simulink model "single_phase_multilevel"  (R2025a)
settings: Solver=ode1be  StartTime=0.0  StopTime=simlength  FixedStep=tc  RelTol=1e-3
values from neighbouring files (symbols this model uses):
  Vfc1_base = Udc/5    [plotting_results.m]    (also in plotting_results_hf.m)
  Vfc2_base = 2*Vfc1_base    [plotting_results.m]    (also in plotting_results_hf.m)
  Vfc3_base = 3*Vfc1_base    [plotting_results.m]    (also in plotting_results_hf.m)
  Vfc4_base = 4*Vfc1_base    [plotting_results.m]    (also in plotting_results_hf.m)
undefined symbols (not defined in the file or in its folder): DThs_init, g0_4Hz, g1_4Hz, I_FS, kalman_omega, kalman_theta, ki_i_inv, ki_v_inv, kp_i_inv, kp_v_inv, Lconn, LFu1, m_dead_time, m_duty_open_loop, magnitude, n1, n10, omega_ref, phase_shift_mod11, phase_shift_mod21, phase_shift_mod31, phase_shift_mod41, phase_shift_mod51, precharge_off, q1kalman, q2kalman, Rbalance, Rconn, RFu, Rg_off, Rg_on, Rkalman, RLFu1, Rprecharge, Tambient, tc, time_pwm_enable, tPWM, ts, V_FS, VCFc_5_init, Vgate_base, weigth
libraries: fl_lib x281, nesl_utility x97, ee_lib x15, simulink x1
(part 4 of 6)

== system single_phase_multilevel/vi_ctrl/modulator1 ==
  m : Inport
  Constant7 : Constant  Value=-m_dead_time
  Constant8 : Constant  Value=m_dead_time
  Data Type Conversion : DataTypeConversion  OutDataTypeStr=double  SaturateOnIntegerOverflow=off  RndMeth=Floor
  Data Type Conversion1 : DataTypeConversion  OutDataTypeStr=double  SaturateOnIntegerOverflow=off  RndMeth=Floor
  Gain : Gain  Gain=Vgate_base
  Gain1 : Gain  Gain=Vgate_base
  Relational Operator : RelationalOperator  Operator=<=
  Relational Operator1 : RelationalOperator  Operator=<=
  Sum1 : Sum  Inputs=|++
  Sum2 : Sum  Inputs=++|
  g11/g12 : Scope  NumInputPorts=2
      settings: SampleTime=tc  ActiveDisplayYMinimum=-0.12499999999999997  ActiveDisplayYMaximum=1.125
  triangle_1 : Subsystem
  g11 : Outport
  g12 : Outport  Port=2
  tag scope: carry_g11=global
  wires:
  m/1 -> Sum1/2, Sum2/1
  Relational Operator/1 -> Data Type Conversion/1
  Relational Operator1/1 -> Data Type Conversion1/1
  Data Type Conversion/1 -> g11/g12/1, Gain/1
  triangle_1/1(carry_mod11) -> Relational Operator1/2, Relational Operator/1, [carry_g11]
  Constant7/1 -> Sum1/1
  Data Type Conversion1/1 -> g11/g12/2, Gain1/1
  Sum2/1 -> Relational Operator1/1
  Constant8/1 -> Sum2/2
  Sum1/1 -> Relational Operator/2
  Gain/1 -> g11/1
  Gain1/1 -> g12/1

== system single_phase_multilevel/vi_ctrl/modulator2 ==
  m : Inport
  Constant7 : Constant  Value=-m_dead_time
  Constant8 : Constant  Value=m_dead_time
  Data Type Conversion : DataTypeConversion  OutDataTypeStr=double  SaturateOnIntegerOverflow=off  RndMeth=Floor
  Data Type Conversion1 : DataTypeConversion  OutDataTypeStr=double  SaturateOnIntegerOverflow=off  RndMeth=Floor
  Gain : Gain  Gain=Vgate_base
  Gain1 : Gain  Gain=Vgate_base
  Relational Operator : RelationalOperator  Operator=<=
  Relational Operator1 : RelationalOperator  Operator=<=
  Sum1 : Sum  Inputs=|++
  Sum2 : Sum  Inputs=++|
  triangle_1 : Subsystem
  g21 : Outport
  g22 : Outport  Port=2
  tag scope: carry_g21=global
  wires:
  Sum1/1 -> Relational Operator/2
  Constant8/1 -> Sum2/2
  Sum2/1 -> Relational Operator1/1
  Data Type Conversion1/1 -> Gain1/1
  Constant7/1 -> Sum1/1
  triangle_1/1(carry_mod21) -> [carry_g21], Relational Operator1/2, Relational Operator/1
  Data Type Conversion/1 -> Gain/1
  Relational Operator1/1 -> Data Type Conversion1/1
  Relational Operator/1 -> Data Type Conversion/1
  m/1 -> Sum2/1, Sum1/2
  Gain/1 -> g21/1
  Gain1/1 -> g22/1

== system single_phase_multilevel/vi_ctrl/modulator3 ==
  m : Inport
  Constant7 : Constant  Value=-m_dead_time
  Constant8 : Constant  Value=m_dead_time
  Data Type Conversion : DataTypeConversion  OutDataTypeStr=double  SaturateOnIntegerOverflow=off  RndMeth=Floor
  Data Type Conversion1 : DataTypeConversion  OutDataTypeStr=double  SaturateOnIntegerOverflow=off  RndMeth=Floor
  Gain : Gain  Gain=Vgate_base
  Gain1 : Gain  Gain=Vgate_base
  Relational Operator : RelationalOperator  Operator=<=
  Relational Operator1 : RelationalOperator  Operator=<=
  Sum1 : Sum  Inputs=|++
  Sum2 : Sum  Inputs=++|
  triangle_1 : Subsystem
  g21 : Outport
  g22 : Outport  Port=2
  tag scope: carry_g31=global
  wires:
  m/1 -> Sum1/2, Sum2/1
  Relational Operator/1 -> Data Type Conversion/1
  Relational Operator1/1 -> Data Type Conversion1/1
  Data Type Conversion/1 -> Gain/1
  triangle_1/1(carry_mod21) -> Relational Operator/1, Relational Operator1/2, [carry_g31]
  Constant7/1 -> Sum1/1
  Data Type Conversion1/1 -> Gain1/1
  Sum2/1 -> Relational Operator1/1
  Constant8/1 -> Sum2/2
  Sum1/1 -> Relational Operator/2
  Gain/1 -> g21/1
  Gain1/1 -> g22/1

== system single_phase_multilevel/vi_ctrl/modulator4 ==
  m : Inport
  Constant7 : Constant  Value=-m_dead_time
  Constant8 : Constant  Value=m_dead_time
  Data Type Conversion : DataTypeConversion  OutDataTypeStr=double  SaturateOnIntegerOverflow=off  RndMeth=Floor
  Data Type Conversion1 : DataTypeConversion  OutDataTypeStr=double  SaturateOnIntegerOverflow=off  RndMeth=Floor
  Gain : Gain  Gain=Vgate_base
  Gain1 : Gain  Gain=Vgate_base
  Relational Operator : RelationalOperator  Operator=<=
  Relational Operator1 : RelationalOperator  Operator=<=
  Sum1 : Sum  Inputs=|++
  Sum2 : Sum  Inputs=++|
  triangle_1 : Subsystem
  g21 : Outport
  g22 : Outport  Port=2
  tag scope: carry_g41=global
  wires:
  m/1 -> Sum1/2, Sum2/1
  Relational Operator/1 -> Data Type Conversion/1
  Relational Operator1/1 -> Data Type Conversion1/1
  Data Type Conversion/1 -> Gain/1
  triangle_1/1(carry_mod21) -> Relational Operator/1, Relational Operator1/2, [carry_g41]
  Constant7/1 -> Sum1/1
  Data Type Conversion1/1 -> Gain1/1
  Sum2/1 -> Relational Operator1/1
  Constant8/1 -> Sum2/2
  Sum1/1 -> Relational Operator/2
  Gain/1 -> g21/1
  Gain1/1 -> g22/1

== system single_phase_multilevel/vi_ctrl/modulator5 ==
  m : Inport
  Constant7 : Constant  Value=-m_dead_time
  Constant8 : Constant  Value=m_dead_time
  Data Type Conversion : DataTypeConversion  OutDataTypeStr=double  SaturateOnIntegerOverflow=off  RndMeth=Floor
  Data Type Conversion1 : DataTypeConversion  OutDataTypeStr=double  SaturateOnIntegerOverflow=off  RndMeth=Floor
  Gain : Gain  Gain=Vgate_base
  Gain1 : Gain  Gain=Vgate_base
  Relational Operator : RelationalOperator  Operator=<=
  Relational Operator1 : RelationalOperator  Operator=<=
  Sum1 : Sum  Inputs=|++
  Sum2 : Sum  Inputs=++|
  triangle_1 : Subsystem
  g21 : Outport
  g22 : Outport  Port=2
  tag scope: carry_g51=global
  wires:
  Sum1/1 -> Relational Operator/2
  Constant8/1 -> Sum2/2
  Sum2/1 -> Relational Operator1/1
  Data Type Conversion1/1 -> Gain1/1
  Constant7/1 -> Sum1/1
  triangle_1/1(carry_mod21) -> [carry_g51], Relational Operator1/2, Relational Operator/1
  Data Type Conversion/1 -> Gain/1
  Relational Operator1/1 -> Data Type Conversion1/1
  Relational Operator/1 -> Data Type Conversion/1
  m/1 -> Sum2/1, Sum1/2
  Gain/1 -> g21/1
  Gain1/1 -> g22/1

== system single_phase_multilevel/vi_ctrl/pre-charge ==
  dm_in : Inport
  Ramp : simulink/Sources/Ramp  slope=-1  start=0  InitialOutput=0.5
  Saturation : Saturate  UpperLimit=0.25  LowerLimit=0
  Step1 : Step  Time=time_pwm_enable  SampleTime=0
  Switch : Switch  Criteria=u2 > Threshold  Threshold=0.5  SaturateOnIntegerOverflow=off  InputSameDT=off
  dm_out : Outport
  wires:
  Switch/1 -> dm_out/1
  ? -> Saturation/1
  Saturation/1 -> Switch/3
  dm_in/1 -> Switch/1
  Step1/1 -> Switch/2

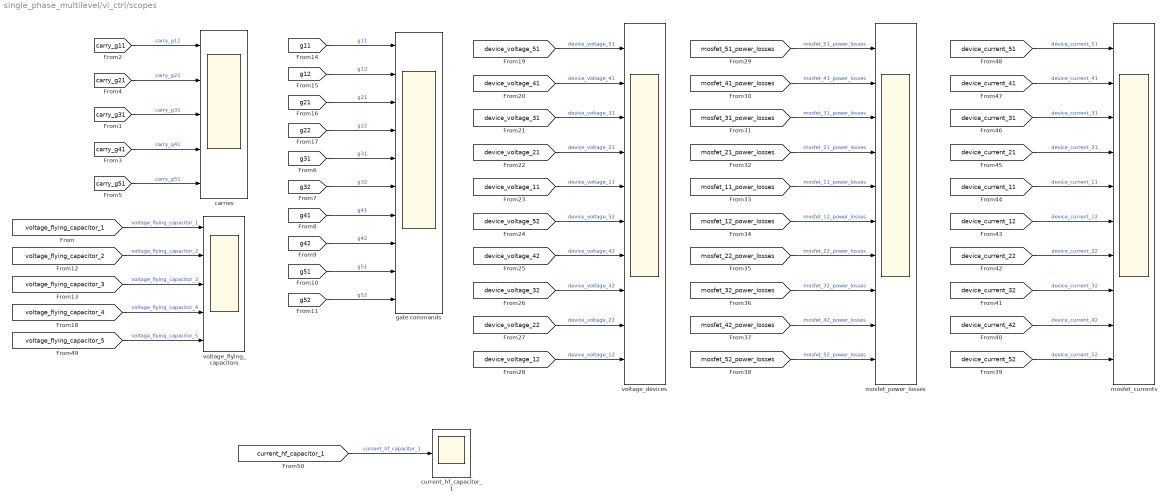
== system single_phase_multilevel/vi_ctrl/scopes ==
  carries : Scope  NumInputPorts=5
      settings: SampleTime=tc  ActiveDisplayYMinimum=-1.64662  ActiveDisplayYMaximum=1.23308  DataLoggingVariableName=ScopeData2
  current_hf_capacitor_1 : Scope
      settings: SampleTime=tc  ActiveDisplayYMinimum=-3.192455025047797  ActiveDisplayYMaximum=2.3538130408116107
  gate commands : Scope  NumInputPorts=10
      settings: SampleTime=tc  ActiveDisplayYMinimum=-1.875  ActiveDisplayYMaximum=16.875  DataLoggingVariableName=ScopeData3
  mosfet_currents : Scope  NumInputPorts=10
      settings: SampleTime=tc  ActiveDisplayYMinimum=-162.1625098340769  ActiveDisplayYMaximum=1459.4625889259892
  mosfet_power_losses : Scope  NumInputPorts=10
      settings: SampleTime=tc  ActiveDisplayYMinimum=-0.01246  ActiveDisplayYMaximum=0.84421  DataLoggingVariableName=ScopeData2
  voltage_devices : Scope  NumInputPorts=10
      settings: SampleTime=tc  ActiveDisplayYMinimum=1.7653686212392756  ActiveDisplayYMaximum=403.40848662720771  DataLoggingVariableName=ScopeData3
  voltage_flying_capacitors : Scope  NumInputPorts=5
      settings: SampleTime=tc  ActiveDisplayYMinimum=-145.59590564608663  ActiveDisplayYMaximum=3675.5801398737103
  wires:
  [carry_g51] -> carries/5  "carry_g51"
  [g12] -> gate commands/2  "g12"
  [g11] -> gate commands/1  "g11"
  [g41] -> gate commands/7  "g41"
  [carry_g41] -> carries/4  "carry_g41"
  [g52] -> gate commands/10  "g52"
  [carry_g31] -> carries/3  "carry_g31"
  [g31] -> gate commands/5  "g31"
  [g21] -> gate commands/3  "g21"
  [voltage_flying_capacitor_4] -> voltage_flying_capacitors/4  "voltage_flying_capacitor_4"
  [carry_g11] -> carries/1  "carry_g11"
  [g42] -> gate commands/8  "g42"
  [voltage_flying_capacitor_1] -> voltage_flying_capacitors/1  "voltage_flying_capacitor_1"
  [g22] -> gate commands/4  "g22"
  [g32] -> gate commands/6  "g32"
  [g51] -> gate commands/9  "g51"
  [voltage_flying_capacitor_3] -> voltage_flying_capacitors/3  "voltage_flying_capacitor_3"
  [voltage_flying_capacitor_2] -> voltage_flying_capacitors/2  "voltage_flying_capacitor_2"
  [carry_g21] -> carries/2  "carry_g21"
  [device_current_11] -> mosfet_currents/5  "device_current_11"
  [mosfet_12_power_losses] -> mosfet_power_losses/6  "mosfet_12_power_losses"
  [device_current_32] -> mosfet_currents/8  "device_current_32"
  [mosfet_21_power_losses] -> mosfet_power_losses/4  "mosfet_21_power_losses"
  [device_voltage_42] -> voltage_devices/7  "device_voltage_42"
  [device_voltage_21] -> voltage_devices/4  "device_voltage_21"
  [device_current_12] -> mosfet_currents/6  "device_current_12"
  [device_voltage_52] -> voltage_devices/6  "device_voltage_52"
  [device_voltage_41] -> voltage_devices/2  "device_voltage_41"
  [device_voltage_51] -> voltage_devices/1  "device_voltage_51"
  [device_voltage_11] -> voltage_devices/5  "device_voltage_11"
  [mosfet_31_power_losses] -> mosfet_power_losses/3  "mosfet_31_power_losses"
  [device_voltage_22] -> voltage_devices/9  "device_voltage_22"
  [device_current_51] -> mosfet_currents/1  "device_current_51"
  [device_current_41] -> mosfet_currents/2  "device_current_41"
  [device_voltage_12] -> voltage_devices/10  "device_voltage_12"
  [device_voltage_32] -> voltage_devices/8  "device_voltage_32"
  [device_voltage_31] -> voltage_devices/3  "device_voltage_31"
  [mosfet_32_power_losses] -> mosfet_power_losses/8  "mosfet_32_power_losses"
  [mosfet_11_power_losses] -> mosfet_power_losses/5  "mosfet_11_power_losses"
  [mosfet_51_power_losses] -> mosfet_power_losses/1  "mosfet_51_power_losses"
  [mosfet_41_power_losses] -> mosfet_power_losses/2  "mosfet_41_power_losses"
  [mosfet_42_power_losses] -> mosfet_power_losses/9  "mosfet_42_power_losses"
  [mosfet_52_power_losses] -> mosfet_power_losses/10  "mosfet_52_power_losses"
  [mosfet_22_power_losses] -> mosfet_power_losses/7  "mosfet_22_power_losses"
  [device_current_42] -> mosfet_currents/9  "device_current_42"
  [device_current_31] -> mosfet_currents/3  "device_current_31"
  [device_current_22] -> mosfet_currents/7  "device_current_22"
  [device_current_21] -> mosfet_currents/4  "device_current_21"
  [device_current_52] -> mosfet_currents/10  "device_current_52"
  [voltage_flying_capacitor_5] -> voltage_flying_capacitors/5  "voltage_flying_capacitor_5"
  [current_hf_capacitor_1] -> current_hf_capacitor_1/1  "current_hf_capacitor_1"

== system single_phase_multilevel/vi_ctrl/single_phase_contrl_system ==
  1/Ti2 : Gain  Gain=1/V_FS  SaturateOnIntegerOverflow=on  OutDataTypeStr=Inherit: Same as input  ParamDataTypeStr=Inherit: Same as input
  Constant1 : Constant  Value=0
  Math Function : Math  Operator=magnitude^2
  Math Function1 : Math  Operator=magnitude^2
  Sqrt : Sqrt
  Sum1 : Sum  Inputs=|-+
  Sum2 : Sum  Inputs=+-|
  Sum3 : Sum  Inputs=|++
  Sum4 : Sum  Inputs=|-+
  Zero-Order Hold4 : ZeroOrderHold  SampleTime=ts
  acquisition_and_scaling_current : Subsystem
  acquisition_and_scaling_voltage : Subsystem
  alpha_beta_transformation_i : Subsystem
  alpha_beta_transformation_v : Subsystem
  alphabeta2dq : Subsystem
  dq2alphabeta : Subsystem
  i_alpha_beta : Scope  NumInputPorts=2
      settings: ActiveDisplayYMinimum=-0.6421  ActiveDisplayYMaximum=0.5039
  idq : Scope  NumInputPorts=2
      settings: ActiveDisplayYMinimum=-0.09367  ActiveDisplayYMaximum=0.50142
  inverter current/voltage : Scope  NumInputPorts=3
      settings: SampleTime=tc  ActiveDisplayYMinimum=-1.0984397723811322E-13  ActiveDisplayYMaximum=2.3609927412802815E-14  DataLoggingVariableName=ScopeData2
  phase_gen : Subsystem
  pi_d : Subsystem
  pi_q : Subsystem
  pi_v : Subsystem
  reference_flt : Subsystem
  v_reference : Step  Time=precharge_off  After=230*sqrt(2)  SampleTime=0
  alpha : Outport
  tag scope: uout_magnitude_pu=global, uout_magnitude_pu_ref=global
  wires:
  [inverter_current_output] -> inverter current/voltage/1  "inverter_current_output_modA"
  [inverter_current_output] -> acquisition_and_scaling_current/1(in)
  pi_d/1(Vd_out) -> dq2alphabeta/1(d)
  pi_v/1(i_ref_internal) -> Sum2/1
  Zero-Order Hold4/1 -> reference_flt/1(input)
  alpha_beta_transformation_v/2(beta) -> Math Function1/1
  [inverter_voltage_output] -> inverter current/voltage/2  "inverter_voltager_output_modA"
  alphabeta2dq/2("q ") -> idq/2, Sum1/1
  dq2alphabeta/1(alpha) -> alpha/1
  [inverter_voltage_output] -> acquisition_and_scaling_voltage/1(in)
  Constant1/1 -> Sum1/2
  alphabeta2dq/1("d ") -> idq/1, Sum2/2
  v_reference/1 -> 1/Ti2/1
  Sum4/1 -> pi_v/1(e)
  Math Function1/1 -> Sum3/2
  phase_gen/1(theta) -> alphabeta2dq/3(wt), dq2alphabeta/3(wt)
  1/Ti2/1 -> Zero-Order Hold4/1
  acquisition_and_scaling_current/1(out) -> alpha_beta_transformation_i/1(in)
  Sum3/1 -> Sqrt/1
  Sum1/1 -> pi_q/1(iq_tilde)
  Math Function/1 -> Sum3/1
  Sqrt/1 -> [uout_magnitude_pu], Sum4/1
  pi_q/1(Vd_out) -> dq2alphabeta/2(q)
  Sum2/1 -> pi_d/1(id_tilde)
  alpha_beta_transformation_i/1(alpha) -> i_alpha_beta/1, alphabeta2dq/1(alpha)
  alpha_beta_transformation_i/2(beta) -> i_alpha_beta/2, alphabeta2dq/2(beta)
  acquisition_and_scaling_voltage/1(out) -> alpha_beta_transformation_v/1(in)
  alpha_beta_transformation_v/1(alpha) -> Math Function/1
  [inverter_current_stack] -> inverter current/voltage/3  "inverter_current_stack_modA"
  reference_flt/1(output) -> [uout_magnitude_pu_ref], Sum4/2

== system single_phase_multilevel/flying_capacitor_leg/switch_11/Subsystem ==
  Diode : fl_lib/Electrical/Electrical Elements/Diode  Vf=Vgamma_diode_mosfet V  Ron=Ron_diode_mosfet Ohm  Goff=1e-8 1/Ohm  i_specify=off  i_priority=None  i=0 A  i_nominal_specify=off  i_nominal_value=1  i_nominal_unit=A  v_specify=off  v_priority=None  v=0 V  v_nominal_specify=off  v_nominal_value=1  v_nominal_unit=V
  G3R160MT17D : ee_lib/Semiconductors & Converters/MOSFET (Ideal, Switching)  port_option=ee.enum.controlport.elec  Rds=Rds_on Ohm  Goff=Goff_state_mosfet 1/Ohm  Vth=Vg_threshold V  diode_param=ee.enum.semiconductors.protectionDiode.external  diode_Vf=Vgamma_diode_mosfet V  diode_Ron=Ron_diode_mosfet Ohm  diode_Goff=Goff_state_mosfet 1/Ohm  diode_C=50e-9 F  diode_iRM=-235 A  diode_iF=300 A  diode_idot=-50 A/us  diode_trr_param=ee.enum.converters.diodeReverseParam.trr_factor  diode_trr_factor=3  diode_trr=15 us  diode_Qrr=1500 s*uA  ids_specify=off  ids_priority=None  ids=0 A  ids_nominal_specify=off  ids_nominal_value=1  ids_nominal_unit=A  vds_specify=off  vds_priority=None  vds=0 V  vds_nominal_specify=off  vds_nominal_value=1  vds_nominal_unit=V  vgs_specify=off  vgs_priority=None  vgs=0 V  vgs_nominal_specify=off  vgs_nominal_value=1  vgs_nominal_unit=V  thermal_loss_option=ee.enum.converters.thermalLossOption.constantvalues  Von_data=[0, 1.8, 3.2, 6, 10, 16; 0, 2, 5.5, 9.5, 15, 25] V  Tj=[298.15, 448.15] K  Iout_data=[0, 20, 40, 60, 80, 100] A  Eon_data=[0, 55.04, 124.57, 235.53, 362.12; 0, 71.25, 161.25, 304.88, 468.75] * 1e-6 J  Eoff_data=[0, 18, 30, 56.1, 76.5; 0, 22.5, 37.5, 70.13, 95.63] * 1e-6 J  Eon_data_3D=[zeros(2, 5, 3)] J  Eoff_data_3D=[zeros(2, 5, 3)] J  Tj_loss=[298.15, 448.15] K  Iout_data_loss=[0, 10, 20, 30, 40] A  tabulateWithVds=false  Vds_loss=[0, 150, 300] V  Eon_scalar=Eon J  Eoff_scalar=Eoff J  Voff=Vdc_switching_losses_ref V  Iout_scalar=Ids_switching_losses_ref A  useCurrentFromPreviousCycle=false  useVoltageFromPreviousCycle=false  diodeModelType=ee.enum.converters.diodeModelType.pwl  diodeTableType=ee.enum.diode.tableType.IfMat  diode_ReverseIVType=ee.enum.diode.diodeReverseIV.constant  diode_IfMat=[.07, .12, .19, 1.75, 4.24, 7.32, 11.2; .16, .3, .72, 2.14, 4.02, 6.35, 9.12] A  diode_VfMat=[.9, 1.15, 1.25, 1.5, 1.75, 2.17, 2.6, 2.85; .58, .68, .75, 1.1, 1.38, 1.77, 2.27, 2.7] V  diode_TjVec=[25, 125] degC  diode_VfVec=[.5, .7, .9, 1.3, 1.7, 2.1, 2.5] V  diode_IfVec=[.1, .2, .5, 1, 2, 4, 7, 10] A  diode_IrMat=[1e-06, 2e-06, 5e-06, 1e-05, 2.5e-05, 5e-05, .0001; 2e-06, 5e-06, 1e-05, 4e-05, 8e-05, .0002, .0005] A  diode_VrMat=[10, 100, 200, 250, 300, 325, 350; 10, 70, 160, 220, 270, 300, 320] V  diode_VrVec=[10, 20, 40, 50, 70, 80, 100] V  diode_IrVec=[1e-06, 2e-06, 5e-06, 1e-05, 2e-05, 5e-05, .0001] A  diode_Vr=-600 V  diode_Ls=150 nH  diode_Erec=0.03 J  diode_rec_loss_model=ee.enum.diode.reverseRecoveryModel.fixed  diode_ErecVal=0 J  diode_scaleWithIandV=true  diode_ErecMat=zeros(2, 3) J  diode_TjrecVec=[298.15, 398.15] K  diode_IfrecVec=[.1, 1, 10] A  diode_IrecVal=10 A  diode_VrecVal=10 V  diode_tFilter=1 / 1000 / 100 s  separateThermalPortForDiode=false  thermal_network_parameterization=ee.enum.thermalNetworkTopology.external  Rth=[.03, .2] K/W  Rth_Cauer=[.03, .1, .2] K/W  Rth_Foster=[.03, .2] K/W  thermal_mass_parameterization=ee.enum.thermalNetwork.timeconstant  thermal_mass=[3, 25] J/K  thermal_mass_Cauer=[3, 10, 25] J/K  thermal_mass_Foster=[33, 50] J/K  thermal_time_constant=[.1, 5] s  thermal_time_constant_Cauer=[.1, 1, 5] s  thermal_time_constant_Foster=[1, 10] s  thermal_mass_initial_temperatures=[25, 25] degC  thermal_mass_initial_temperatures_Cauer=[25, 25, 25] degC  junction_thermal_mass=JunctionTermalMass J/K  Tvec_initial_Foster=[25, 25, 25, 25] degC  RthDiode=[.03, .2] K/W  RthCauerDiode=[.03, .1, .2] K/W  RthFosterDiode=[.03, .2] K/W  thermalMassDiode=[3, 25] J/K  thermalMassCauerDiode=[3, 10, 25] J/K  thermalMassFosterDiode=[33, 50] J/K  thermalTauDiode=[.1, 5] s  thermalTauCauerDiode=[.1, 1, 5] s  thermalTauFosterDiode=[1, 10] s  thermalMassInitTempDiode=[25, 25] degC  thermalMassInitTempCauerDiode=[25, 25, 25] degC  junctionthermalMassDiode=0.1 J/K  TVecInitialFosterDiode=[25, 25, 25, 25] degC  no_thermal_network=0  mosfet_junction_temperature_specify=off  mosfet_junction_temperature_priority=None  mosfet_junction_temperature=25 degC  mosfet_junction_temperature_nominal_specify=off  mosfet_junction_temperature_nominal_value=1  mosfet_junction_temperature_nominal_unit=degC  diode_junction_temperature_specify=off  diode_junction_temperature_priority=None  diode_junction_temperature=25 degC  diode_junction_temperature_nominal_specify=off  diode_junction_temperature_nominal_value=1  diode_junction_temperature_nominal_unit=degC  Qj_specify=off  Qj_priority=None  Qj=0 W  Qj_nominal_specify=off  Qj_nominal_value=1  Qj_nominal_unit=W  accumulatedSwitchingLosses_specify=off  accumulatedSwitchingLosses_priority=None  accumulatedSwitchingLosses=0 J
      settings: InternalSimscapePortConfiguration="{\"Bottom\":[],\"Left\":[{\"id\":\"G_elec\",\"label\":\"\",\"type\":\"foundation.electrical.electrical\"},{\"id\":\"H\",\"label\":\"\",\"type\":\"foundation.thermal.thermal\"}],\"Right\":[{\"id\":\"D\",\"label\":\"\",\"type\":\"foundation.electrical.electrical\"},{\"id\":\"S\",\"label\":\"\",\"type\":\"foundation.electrical.electrical\"}],\"Top\":[]}"
  G : PMIOPort  Side=Left
  thermal_port : PMIOPort  Port=2  Side=Left
  D : PMIOPort  Port=3  Side=Left
  S : PMIOPort  Port=4  Side=Right
  connections:
  G3R160MT17D/RConn1 -- Diode/RConn1 -- D/RConn1
  G3R160MT17D/RConn2 -- Diode/LConn1 -- S/RConn1
  G/RConn1 -- G3R160MT17D/LConn1
  G3R160MT17D/LConn2 -- thermal_port/RConn1

== system single_phase_multilevel/flying_capacitor_leg/switch_11/gate_driver ==
  cmd : Inport
  Controlled Voltage Source : fl_lib/Electrical/Electrical Sources/Controlled Voltage Source
  Diode1 : fl_lib/Electrical/Electrical Elements/Diode  Vf=0.6 V  Ron=0.3 Ohm  Goff=1e-8 1/Ohm  i_specify=off  i_priority=None  i=0 A  i_nominal_specify=off  i_nominal_value=1  i_nominal_unit=A  v_specify=off  v_priority=None  v=0 V  v_nominal_specify=off  v_nominal_value=1  v_nominal_unit=V
  Diode2 : fl_lib/Electrical/Electrical Elements/Diode  Vf=0.6 V  Ron=0.3 Ohm  Goff=1e-8 1/Ohm  i_specify=off  i_priority=None  i=0 A  i_nominal_specify=off  i_nominal_value=1  i_nominal_unit=A  v_specify=off  v_priority=None  v=0 V  v_nominal_specify=off  v_nominal_value=1  v_nominal_unit=V
  Resistor : fl_lib/Electrical/Electrical Elements/Resistor  R=Rg_on Ohm  i_specify=off  i_priority=None  i=0 A  i_nominal_specify=off  i_nominal_value=1  i_nominal_unit=A  v_specify=off  v_priority=None  v=0 V  v_nominal_specify=off  v_nominal_value=1  v_nominal_unit=V
  Resistor1 : fl_lib/Electrical/Electrical Elements/Resistor  R=Rg_off Ohm  i_specify=off  i_priority=None  i=0 A  i_nominal_specify=off  i_nominal_value=1  i_nominal_unit=A  v_specify=off  v_priority=None  v=0 V  v_nominal_specify=off  v_nominal_value=1  v_nominal_unit=V
  Simulink-PS Converter : nesl_utility/Simulink-PS Converter  PhysicalDomain=network_engine_domain  SubClassName=ps_input  LeftPortType=input  RightPortType=output  PseudoPeriodic=off  Frequencies=[]  NoiseDistribution=none  NoiseParameters=[]  Unit=V  AffineConversion=off  FilteringAndDerivatives=provide  SimscapeFilterOrder=1  InputFilterTimeConstant=0.001  UdotUserProvided=0
  gate : PMIOPort  Side=Right
  source : PMIOPort  Port=2  Side=Right
  wires:
  cmd/1 -> Simulink-PS Converter/1
  connections:
  Resistor/LConn1 -- Controlled Voltage Source/LConn1 -- Resistor1/LConn1
  Diode2/LConn1 -- Resistor/RConn1
  Controlled Voltage Source/RConn1 -- Simulink-PS Converter/RConn1
  Controlled Voltage Source/RConn2 -- source/RConn1
  Diode1/LConn1 -- gate/RConn1 -- Diode2/RConn1
  Diode1/RConn1 -- Resistor1/RConn1

== system single_phase_multilevel/flying_capacitor_leg/switch_12/Subsystem ==
  Diode : fl_lib/Electrical/Electrical Elements/Diode  Vf=Vgamma_diode_mosfet V  Ron=Ron_diode_mosfet Ohm  Goff=1e-8 1/Ohm  i_specify=off  i_priority=None  i=0 A  i_nominal_specify=off  i_nominal_value=1  i_nominal_unit=A  v_specify=off  v_priority=None  v=0 V  v_nominal_specify=off  v_nominal_value=1  v_nominal_unit=V
  G3R160MT17D : ee_lib/Semiconductors & Converters/MOSFET (Ideal, Switching)  port_option=ee.enum.controlport.elec  Rds=Rds_on Ohm  Goff=Goff_state_mosfet 1/Ohm  Vth=Vg_threshold V  diode_param=ee.enum.semiconductors.protectionDiode.external  diode_Vf=Vgamma_diode_mosfet V  diode_Ron=Ron_diode_mosfet Ohm  diode_Goff=Goff_state_mosfet 1/Ohm  diode_C=50e-9 F  diode_iRM=-235 A  diode_iF=300 A  diode_idot=-50 A/us  diode_trr_param=ee.enum.converters.diodeReverseParam.trr_factor  diode_trr_factor=3  diode_trr=15 us  diode_Qrr=1500 s*uA  ids_specify=off  ids_priority=None  ids=0 A  ids_nominal_specify=off  ids_nominal_value=1  ids_nominal_unit=A  vds_specify=off  vds_priority=None  vds=0 V  vds_nominal_specify=off  vds_nominal_value=1  vds_nominal_unit=V  vgs_specify=off  vgs_priority=None  vgs=0 V  vgs_nominal_specify=off  vgs_nominal_value=1  vgs_nominal_unit=V  thermal_loss_option=ee.enum.converters.thermalLossOption.constantvalues  Von_data=[0, 1.8, 3.2, 6, 10, 16; 0, 2, 5.5, 9.5, 15, 25] V  Tj=[298.15, 448.15] K  Iout_data=[0, 20, 40, 60, 80, 100] A  Eon_data=[0, 55.04, 124.57, 235.53, 362.12; 0, 71.25, 161.25, 304.88, 468.75] * 1e-6 J  Eoff_data=[0, 18, 30, 56.1, 76.5; 0, 22.5, 37.5, 70.13, 95.63] * 1e-6 J  Eon_data_3D=[zeros(2, 5, 3)] J  Eoff_data_3D=[zeros(2, 5, 3)] J  Tj_loss=[298.15, 448.15] K  Iout_data_loss=[0, 10, 20, 30, 40] A  tabulateWithVds=false  Vds_loss=[0, 150, 300] V  Eon_scalar=Eon J  Eoff_scalar=Eoff J  Voff=Vdc_switching_losses_ref V  Iout_scalar=Ids_switching_losses_ref A  useCurrentFromPreviousCycle=false  useVoltageFromPreviousCycle=false  diodeModelType=ee.enum.converters.diodeModelType.pwl  diodeTableType=ee.enum.diode.tableType.IfMat  diode_ReverseIVType=ee.enum.diode.diodeReverseIV.constant  diode_IfMat=[.07, .12, .19, 1.75, 4.24, 7.32, 11.2; .16, .3, .72, 2.14, 4.02, 6.35, 9.12] A  diode_VfMat=[.9, 1.15, 1.25, 1.5, 1.75, 2.17, 2.6, 2.85; .58, .68, .75, 1.1, 1.38, 1.77, 2.27, 2.7] V  diode_TjVec=[25, 125] degC  diode_VfVec=[.5, .7, .9, 1.3, 1.7, 2.1, 2.5] V  diode_IfVec=[.1, .2, .5, 1, 2, 4, 7, 10] A  diode_IrMat=[1e-06, 2e-06, 5e-06, 1e-05, 2.5e-05, 5e-05, .0001; 2e-06, 5e-06, 1e-05, 4e-05, 8e-05, .0002, .0005] A  diode_VrMat=[10, 100, 200, 250, 300, 325, 350; 10, 70, 160, 220, 270, 300, 320] V  diode_VrVec=[10, 20, 40, 50, 70, 80, 100] V  diode_IrVec=[1e-06, 2e-06, 5e-06, 1e-05, 2e-05, 5e-05, .0001] A  diode_Vr=-600 V  diode_Ls=150 nH  diode_Erec=0.03 J  diode_rec_loss_model=ee.enum.diode.reverseRecoveryModel.fixed  diode_ErecVal=0 J  diode_scaleWithIandV=true  diode_ErecMat=zeros(2, 3) J  diode_TjrecVec=[298.15, 398.15] K  diode_IfrecVec=[.1, 1, 10] A  diode_IrecVal=10 A  diode_VrecVal=10 V  diode_tFilter=1 / 1000 / 100 s  separateThermalPortForDiode=false  thermal_network_parameterization=ee.enum.thermalNetworkTopology.external  Rth=[.03, .2] K/W  Rth_Cauer=[.03, .1, .2] K/W  Rth_Foster=[.03, .2] K/W  thermal_mass_parameterization=ee.enum.thermalNetwork.timeconstant  thermal_mass=[3, 25] J/K  thermal_mass_Cauer=[3, 10, 25] J/K  thermal_mass_Foster=[33, 50] J/K  thermal_time_constant=[.1, 5] s  thermal_time_constant_Cauer=[.1, 1, 5] s  thermal_time_constant_Foster=[1, 10] s  thermal_mass_initial_temperatures=[25, 25] degC  thermal_mass_initial_temperatures_Cauer=[25, 25, 25] degC  junction_thermal_mass=JunctionTermalMass J/K  Tvec_initial_Foster=[25, 25, 25, 25] degC  RthDiode=[.03, .2] K/W  RthCauerDiode=[.03, .1, .2] K/W  RthFosterDiode=[.03, .2] K/W  thermalMassDiode=[3, 25] J/K  thermalMassCauerDiode=[3, 10, 25] J/K  thermalMassFosterDiode=[33, 50] J/K  thermalTauDiode=[.1, 5] s  thermalTauCauerDiode=[.1, 1, 5] s  thermalTauFosterDiode=[1, 10] s  thermalMassInitTempDiode=[25, 25] degC  thermalMassInitTempCauerDiode=[25, 25, 25] degC  junctionthermalMassDiode=0.1 J/K  TVecInitialFosterDiode=[25, 25, 25, 25] degC  no_thermal_network=0  mosfet_junction_temperature_specify=off  mosfet_junction_temperature_priority=None  mosfet_junction_temperature=25 degC  mosfet_junction_temperature_nominal_specify=off  mosfet_junction_temperature_nominal_value=1  mosfet_junction_temperature_nominal_unit=degC  diode_junction_temperature_specify=off  diode_junction_temperature_priority=None  diode_junction_temperature=25 degC  diode_junction_temperature_nominal_specify=off  diode_junction_temperature_nominal_value=1  diode_junction_temperature_nominal_unit=degC  Qj_specify=off  Qj_priority=None  Qj=0 W  Qj_nominal_specify=off  Qj_nominal_value=1  Qj_nominal_unit=W  accumulatedSwitchingLosses_specify=off  accumulatedSwitchingLosses_priority=None  accumulatedSwitchingLosses=0 J
      settings: InternalSimscapePortConfiguration="{\"Bottom\":[],\"Left\":[{\"id\":\"G_elec\",\"label\":\"\",\"type\":\"foundation.electrical.electrical\"},{\"id\":\"H\",\"label\":\"\",\"type\":\"foundation.thermal.thermal\"}],\"Right\":[{\"id\":\"D\",\"label\":\"\",\"type\":\"foundation.electrical.electrical\"},{\"id\":\"S\",\"label\":\"\",\"type\":\"foundation.electrical.electrical\"}],\"Top\":[]}"
  G : PMIOPort  Side=Left
  thermal_port : PMIOPort  Port=2  Side=Left
  D : PMIOPort  Port=3  Side=Left
  S : PMIOPort  Port=4  Side=Right
  connections:
  G3R160MT17D/RConn1 -- Diode/RConn1 -- D/RConn1
  G3R160MT17D/RConn2 -- Diode/LConn1 -- S/RConn1
  G/RConn1 -- G3R160MT17D/LConn1
  G3R160MT17D/LConn2 -- thermal_port/RConn1

== system single_phase_multilevel/flying_capacitor_leg/switch_12/gate_driver ==
  cmd : Inport
  Controlled Voltage Source : fl_lib/Electrical/Electrical Sources/Controlled Voltage Source
  Diode1 : fl_lib/Electrical/Electrical Elements/Diode  Vf=0.6 V  Ron=0.3 Ohm  Goff=1e-8 1/Ohm  i_specify=off  i_priority=None  i=0 A  i_nominal_specify=off  i_nominal_value=1  i_nominal_unit=A  v_specify=off  v_priority=None  v=0 V  v_nominal_specify=off  v_nominal_value=1  v_nominal_unit=V
  Diode2 : fl_lib/Electrical/Electrical Elements/Diode  Vf=0.6 V  Ron=0.3 Ohm  Goff=1e-8 1/Ohm  i_specify=off  i_priority=None  i=0 A  i_nominal_specify=off  i_nominal_value=1  i_nominal_unit=A  v_specify=off  v_priority=None  v=0 V  v_nominal_specify=off  v_nominal_value=1  v_nominal_unit=V
  Resistor : fl_lib/Electrical/Electrical Elements/Resistor  R=Rg_on Ohm  i_specify=off  i_priority=None  i=0 A  i_nominal_specify=off  i_nominal_value=1  i_nominal_unit=A  v_specify=off  v_priority=None  v=0 V  v_nominal_specify=off  v_nominal_value=1  v_nominal_unit=V
  Resistor1 : fl_lib/Electrical/Electrical Elements/Resistor  R=Rg_off Ohm  i_specify=off  i_priority=None  i=0 A  i_nominal_specify=off  i_nominal_value=1  i_nominal_unit=A  v_specify=off  v_priority=None  v=0 V  v_nominal_specify=off  v_nominal_value=1  v_nominal_unit=V
  Simulink-PS Converter : nesl_utility/Simulink-PS Converter  PhysicalDomain=network_engine_domain  SubClassName=ps_input  LeftPortType=input  RightPortType=output  PseudoPeriodic=off  Frequencies=[]  NoiseDistribution=none  NoiseParameters=[]  Unit=V  AffineConversion=off  FilteringAndDerivatives=provide  SimscapeFilterOrder=1  InputFilterTimeConstant=0.001  UdotUserProvided=0
  gate : PMIOPort  Side=Right
  source : PMIOPort  Port=2  Side=Right
  wires:
  cmd/1 -> Simulink-PS Converter/1
  connections:
  Resistor/LConn1 -- Controlled Voltage Source/LConn1 -- Resistor1/LConn1
  Diode2/LConn1 -- Resistor/RConn1
  Controlled Voltage Source/RConn1 -- Simulink-PS Converter/RConn1
  Controlled Voltage Source/RConn2 -- source/RConn1
  Diode1/LConn1 -- gate/RConn1 -- Diode2/RConn1
  Diode1/RConn1 -- Resistor1/RConn1

== system single_phase_multilevel/flying_capacitor_leg/switch_21/Subsystem ==
  Diode : fl_lib/Electrical/Electrical Elements/Diode  Vf=Vgamma_diode_mosfet V  Ron=Ron_diode_mosfet Ohm  Goff=1e-8 1/Ohm  i_specify=off  i_priority=None  i=0 A  i_nominal_specify=off  i_nominal_value=1  i_nominal_unit=A  v_specify=off  v_priority=None  v=0 V  v_nominal_specify=off  v_nominal_value=1  v_nominal_unit=V
  G3R160MT17D : ee_lib/Semiconductors & Converters/MOSFET (Ideal, Switching)  port_option=ee.enum.controlport.elec  Rds=Rds_on Ohm  Goff=Goff_state_mosfet 1/Ohm  Vth=Vg_threshold V  diode_param=ee.enum.semiconductors.protectionDiode.external  diode_Vf=Vgamma_diode_mosfet V  diode_Ron=Ron_diode_mosfet Ohm  diode_Goff=Goff_state_mosfet 1/Ohm  diode_C=50e-9 F  diode_iRM=-235 A  diode_iF=300 A  diode_idot=-50 A/us  diode_trr_param=ee.enum.converters.diodeReverseParam.trr_factor  diode_trr_factor=3  diode_trr=15 us  diode_Qrr=1500 s*uA  ids_specify=off  ids_priority=None  ids=0 A  ids_nominal_specify=off  ids_nominal_value=1  ids_nominal_unit=A  vds_specify=off  vds_priority=None  vds=0 V  vds_nominal_specify=off  vds_nominal_value=1  vds_nominal_unit=V  vgs_specify=off  vgs_priority=None  vgs=0 V  vgs_nominal_specify=off  vgs_nominal_value=1  vgs_nominal_unit=V  thermal_loss_option=ee.enum.converters.thermalLossOption.constantvalues  Von_data=[0, 1.8, 3.2, 6, 10, 16; 0, 2, 5.5, 9.5, 15, 25] V  Tj=[298.15, 448.15] K  Iout_data=[0, 20, 40, 60, 80, 100] A  Eon_data=[0, 55.04, 124.57, 235.53, 362.12; 0, 71.25, 161.25, 304.88, 468.75] * 1e-6 J  Eoff_data=[0, 18, 30, 56.1, 76.5; 0, 22.5, 37.5, 70.13, 95.63] * 1e-6 J  Eon_data_3D=[zeros(2, 5, 3)] J  Eoff_data_3D=[zeros(2, 5, 3)] J  Tj_loss=[298.15, 448.15] K  Iout_data_loss=[0, 10, 20, 30, 40] A  tabulateWithVds=false  Vds_loss=[0, 150, 300] V  Eon_scalar=Eon J  Eoff_scalar=Eoff J  Voff=Vdc_switching_losses_ref V  Iout_scalar=Ids_switching_losses_ref A  useCurrentFromPreviousCycle=false  useVoltageFromPreviousCycle=false  diodeModelType=ee.enum.converters.diodeModelType.pwl  diodeTableType=ee.enum.diode.tableType.IfMat  diode_ReverseIVType=ee.enum.diode.diodeReverseIV.constant  diode_IfMat=[.07, .12, .19, 1.75, 4.24, 7.32, 11.2; .16, .3, .72, 2.14, 4.02, 6.35, 9.12] A  diode_VfMat=[.9, 1.15, 1.25, 1.5, 1.75, 2.17, 2.6, 2.85; .58, .68, .75, 1.1, 1.38, 1.77, 2.27, 2.7] V  diode_TjVec=[25, 125] degC  diode_VfVec=[.5, .7, .9, 1.3, 1.7, 2.1, 2.5] V  diode_IfVec=[.1, .2, .5, 1, 2, 4, 7, 10] A  diode_IrMat=[1e-06, 2e-06, 5e-06, 1e-05, 2.5e-05, 5e-05, .0001; 2e-06, 5e-06, 1e-05, 4e-05, 8e-05, .0002, .0005] A  diode_VrMat=[10, 100, 200, 250, 300, 325, 350; 10, 70, 160, 220, 270, 300, 320] V  diode_VrVec=[10, 20, 40, 50, 70, 80, 100] V  diode_IrVec=[1e-06, 2e-06, 5e-06, 1e-05, 2e-05, 5e-05, .0001] A  diode_Vr=-600 V  diode_Ls=150 nH  diode_Erec=0.03 J  diode_rec_loss_model=ee.enum.diode.reverseRecoveryModel.fixed  diode_ErecVal=0 J  diode_scaleWithIandV=true  diode_ErecMat=zeros(2, 3) J  diode_TjrecVec=[298.15, 398.15] K  diode_IfrecVec=[.1, 1, 10] A  diode_IrecVal=10 A  diode_VrecVal=10 V  diode_tFilter=1 / 1000 / 100 s  separateThermalPortForDiode=false  thermal_network_parameterization=ee.enum.thermalNetworkTopology.external  Rth=[.03, .2] K/W  Rth_Cauer=[.03, .1, .2] K/W  Rth_Foster=[.03, .2] K/W  thermal_mass_parameterization=ee.enum.thermalNetwork.timeconstant  thermal_mass=[3, 25] J/K  thermal_mass_Cauer=[3, 10, 25] J/K  thermal_mass_Foster=[33, 50] J/K  thermal_time_constant=[.1, 5] s  thermal_time_constant_Cauer=[.1, 1, 5] s  thermal_time_constant_Foster=[1, 10] s  thermal_mass_initial_temperatures=[25, 25] degC  thermal_mass_initial_temperatures_Cauer=[25, 25, 25] degC  junction_thermal_mass=JunctionTermalMass J/K  Tvec_initial_Foster=[25, 25, 25, 25] degC  RthDiode=[.03, .2] K/W  RthCauerDiode=[.03, .1, .2] K/W  RthFosterDiode=[.03, .2] K/W  thermalMassDiode=[3, 25] J/K  thermalMassCauerDiode=[3, 10, 25] J/K  thermalMassFosterDiode=[33, 50] J/K  thermalTauDiode=[.1, 5] s  thermalTauCauerDiode=[.1, 1, 5] s  thermalTauFosterDiode=[1, 10] s  thermalMassInitTempDiode=[25, 25] degC  thermalMassInitTempCauerDiode=[25, 25, 25] degC  junctionthermalMassDiode=0.1 J/K  TVecInitialFosterDiode=[25, 25, 25, 25] degC  no_thermal_network=0  mosfet_junction_temperature_specify=off  mosfet_junction_temperature_priority=None  mosfet_junction_temperature=25 degC  mosfet_junction_temperature_nominal_specify=off  mosfet_junction_temperature_nominal_value=1  mosfet_junction_temperature_nominal_unit=degC  diode_junction_temperature_specify=off  diode_junction_temperature_priority=None  diode_junction_temperature=25 degC  diode_junction_temperature_nominal_specify=off  diode_junction_temperature_nominal_value=1  diode_junction_temperature_nominal_unit=degC  Qj_specify=off  Qj_priority=None  Qj=0 W  Qj_nominal_specify=off  Qj_nominal_value=1  Qj_nominal_unit=W  accumulatedSwitchingLosses_specify=off  accumulatedSwitchingLosses_priority=None  accumulatedSwitchingLosses=0 J
      settings: InternalSimscapePortConfiguration="{\"Bottom\":[],\"Left\":[{\"id\":\"G_elec\",\"label\":\"\",\"type\":\"foundation.electrical.electrical\"},{\"id\":\"H\",\"label\":\"\",\"type\":\"foundation.thermal.thermal\"}],\"Right\":[{\"id\":\"D\",\"label\":\"\",\"type\":\"foundation.electrical.electrical\"},{\"id\":\"S\",\"label\":\"\",\"type\":\"foundation.electrical.electrical\"}],\"Top\":[]}"
  G : PMIOPort  Side=Left
  thermal_port : PMIOPort  Port=2  Side=Left
  D : PMIOPort  Port=3  Side=Left
  S : PMIOPort  Port=4  Side=Right
  connections:
  G3R160MT17D/RConn1 -- Diode/RConn1 -- D/RConn1
  G3R160MT17D/RConn2 -- Diode/LConn1 -- S/RConn1
  G/RConn1 -- G3R160MT17D/LConn1
  G3R160MT17D/LConn2 -- thermal_port/RConn1

== system single_phase_multilevel/flying_capacitor_leg/switch_21/gate_driver ==
  cmd : Inport
  Controlled Voltage Source : fl_lib/Electrical/Electrical Sources/Controlled Voltage Source
  Diode1 : fl_lib/Electrical/Electrical Elements/Diode  Vf=0.6 V  Ron=0.3 Ohm  Goff=1e-8 1/Ohm  i_specify=off  i_priority=None  i=0 A  i_nominal_specify=off  i_nominal_value=1  i_nominal_unit=A  v_specify=off  v_priority=None  v=0 V  v_nominal_specify=off  v_nominal_value=1  v_nominal_unit=V
  Diode2 : fl_lib/Electrical/Electrical Elements/Diode  Vf=0.6 V  Ron=0.3 Ohm  Goff=1e-8 1/Ohm  i_specify=off  i_priority=None  i=0 A  i_nominal_specify=off  i_nominal_value=1  i_nominal_unit=A  v_specify=off  v_priority=None  v=0 V  v_nominal_specify=off  v_nominal_value=1  v_nominal_unit=V
  Resistor : fl_lib/Electrical/Electrical Elements/Resistor  R=Rg_on Ohm  i_specify=off  i_priority=None  i=0 A  i_nominal_specify=off  i_nominal_value=1  i_nominal_unit=A  v_specify=off  v_priority=None  v=0 V  v_nominal_specify=off  v_nominal_value=1  v_nominal_unit=V
  Resistor1 : fl_lib/Electrical/Electrical Elements/Resistor  R=Rg_off Ohm  i_specify=off  i_priority=None  i=0 A  i_nominal_specify=off  i_nominal_value=1  i_nominal_unit=A  v_specify=off  v_priority=None  v=0 V  v_nominal_specify=off  v_nominal_value=1  v_nominal_unit=V
  Simulink-PS Converter : nesl_utility/Simulink-PS Converter  PhysicalDomain=network_engine_domain  SubClassName=ps_input  LeftPortType=input  RightPortType=output  PseudoPeriodic=off  Frequencies=[]  NoiseDistribution=none  NoiseParameters=[]  Unit=V  AffineConversion=off  FilteringAndDerivatives=provide  SimscapeFilterOrder=1  InputFilterTimeConstant=0.001  UdotUserProvided=0
  gate : PMIOPort  Side=Right
  source : PMIOPort  Port=2  Side=Right
  wires:
  cmd/1 -> Simulink-PS Converter/1
  connections:
  Resistor/LConn1 -- Controlled Voltage Source/LConn1 -- Resistor1/LConn1
  Diode2/LConn1 -- Resistor/RConn1
  Controlled Voltage Source/RConn1 -- Simulink-PS Converter/RConn1
  Controlled Voltage Source/RConn2 -- source/RConn1
  Diode1/LConn1 -- gate/RConn1 -- Diode2/RConn1
  Diode1/RConn1 -- Resistor1/RConn1

== system single_phase_multilevel/flying_capacitor_leg/switch_22/Subsystem ==
  Diode : fl_lib/Electrical/Electrical Elements/Diode  Vf=Vgamma_diode_mosfet V  Ron=Ron_diode_mosfet Ohm  Goff=1e-8 1/Ohm  i_specify=off  i_priority=None  i=0 A  i_nominal_specify=off  i_nominal_value=1  i_nominal_unit=A  v_specify=off  v_priority=None  v=0 V  v_nominal_specify=off  v_nominal_value=1  v_nominal_unit=V
  G3R160MT17D : ee_lib/Semiconductors & Converters/MOSFET (Ideal, Switching)  port_option=ee.enum.controlport.elec  Rds=Rds_on Ohm  Goff=Goff_state_mosfet 1/Ohm  Vth=Vg_threshold V  diode_param=ee.enum.semiconductors.protectionDiode.external  diode_Vf=Vgamma_diode_mosfet V  diode_Ron=Ron_diode_mosfet Ohm  diode_Goff=Goff_state_mosfet 1/Ohm  diode_C=50e-9 F  diode_iRM=-235 A  diode_iF=300 A  diode_idot=-50 A/us  diode_trr_param=ee.enum.converters.diodeReverseParam.trr_factor  diode_trr_factor=3  diode_trr=15 us  diode_Qrr=1500 s*uA  ids_specify=off  ids_priority=None  ids=0 A  ids_nominal_specify=off  ids_nominal_value=1  ids_nominal_unit=A  vds_specify=off  vds_priority=None  vds=0 V  vds_nominal_specify=off  vds_nominal_value=1  vds_nominal_unit=V  vgs_specify=off  vgs_priority=None  vgs=0 V  vgs_nominal_specify=off  vgs_nominal_value=1  vgs_nominal_unit=V  thermal_loss_option=ee.enum.converters.thermalLossOption.constantvalues  Von_data=[0, 1.8, 3.2, 6, 10, 16; 0, 2, 5.5, 9.5, 15, 25] V  Tj=[298.15, 448.15] K  Iout_data=[0, 20, 40, 60, 80, 100] A  Eon_data=[0, 55.04, 124.57, 235.53, 362.12; 0, 71.25, 161.25, 304.88, 468.75] * 1e-6 J  Eoff_data=[0, 18, 30, 56.1, 76.5; 0, 22.5, 37.5, 70.13, 95.63] * 1e-6 J  Eon_data_3D=[zeros(2, 5, 3)] J  Eoff_data_3D=[zeros(2, 5, 3)] J  Tj_loss=[298.15, 448.15] K  Iout_data_loss=[0, 10, 20, 30, 40] A  tabulateWithVds=false  Vds_loss=[0, 150, 300] V  Eon_scalar=Eon J  Eoff_scalar=Eoff J  Voff=Vdc_switching_losses_ref V  Iout_scalar=Ids_switching_losses_ref A  useCurrentFromPreviousCycle=false  useVoltageFromPreviousCycle=false  diodeModelType=ee.enum.converters.diodeModelType.pwl  diodeTableType=ee.enum.diode.tableType.IfMat  diode_ReverseIVType=ee.enum.diode.diodeReverseIV.constant  diode_IfMat=[.07, .12, .19, 1.75, 4.24, 7.32, 11.2; .16, .3, .72, 2.14, 4.02, 6.35, 9.12] A  diode_VfMat=[.9, 1.15, 1.25, 1.5, 1.75, 2.17, 2.6, 2.85; .58, .68, .75, 1.1, 1.38, 1.77, 2.27, 2.7] V  diode_TjVec=[25, 125] degC  diode_VfVec=[.5, .7, .9, 1.3, 1.7, 2.1, 2.5] V  diode_IfVec=[.1, .2, .5, 1, 2, 4, 7, 10] A  diode_IrMat=[1e-06, 2e-06, 5e-06, 1e-05, 2.5e-05, 5e-05, .0001; 2e-06, 5e-06, 1e-05, 4e-05, 8e-05, .0002, .0005] A  diode_VrMat=[10, 100, 200, 250, 300, 325, 350; 10, 70, 160, 220, 270, 300, 320] V  diode_VrVec=[10, 20, 40, 50, 70, 80, 100] V  diode_IrVec=[1e-06, 2e-06, 5e-06, 1e-05, 2e-05, 5e-05, .0001] A  diode_Vr=-600 V  diode_Ls=150 nH  diode_Erec=0.03 J  diode_rec_loss_model=ee.enum.diode.reverseRecoveryModel.fixed  diode_ErecVal=0 J  diode_scaleWithIandV=true  diode_ErecMat=zeros(2, 3) J  diode_TjrecVec=[298.15, 398.15] K  diode_IfrecVec=[.1, 1, 10] A  diode_IrecVal=10 A  diode_VrecVal=10 V  diode_tFilter=1 / 1000 / 100 s  separateThermalPortForDiode=false  thermal_network_parameterization=ee.enum.thermalNetworkTopology.external  Rth=[.03, .2] K/W  Rth_Cauer=[.03, .1, .2] K/W  Rth_Foster=[.03, .2] K/W  thermal_mass_parameterization=ee.enum.thermalNetwork.timeconstant  thermal_mass=[3, 25] J/K  thermal_mass_Cauer=[3, 10, 25] J/K  thermal_mass_Foster=[33, 50] J/K  thermal_time_constant=[.1, 5] s  thermal_time_constant_Cauer=[.1, 1, 5] s  thermal_time_constant_Foster=[1, 10] s  thermal_mass_initial_temperatures=[25, 25] degC  thermal_mass_initial_temperatures_Cauer=[25, 25, 25] degC  junction_thermal_mass=JunctionTermalMass J/K  Tvec_initial_Foster=[25, 25, 25, 25] degC  RthDiode=[.03, .2] K/W  RthCauerDiode=[.03, .1, .2] K/W  RthFosterDiode=[.03, .2] K/W  thermalMassDiode=[3, 25] J/K  thermalMassCauerDiode=[3, 10, 25] J/K  thermalMassFosterDiode=[33, 50] J/K  thermalTauDiode=[.1, 5] s  thermalTauCauerDiode=[.1, 1, 5] s  thermalTauFosterDiode=[1, 10] s  thermalMassInitTempDiode=[25, 25] degC  thermalMassInitTempCauerDiode=[25, 25, 25] degC  junctionthermalMassDiode=0.1 J/K  TVecInitialFosterDiode=[25, 25, 25, 25] degC  no_thermal_network=0  mosfet_junction_temperature_specify=off  mosfet_junction_temperature_priority=None  mosfet_junction_temperature=25 degC  mosfet_junction_temperature_nominal_specify=off  mosfet_junction_temperature_nominal_value=1  mosfet_junction_temperature_nominal_unit=degC  diode_junction_temperature_specify=off  diode_junction_temperature_priority=None  diode_junction_temperature=25 degC  diode_junction_temperature_nominal_specify=off  diode_junction_temperature_nominal_value=1  diode_junction_temperature_nominal_unit=degC  Qj_specify=off  Qj_priority=None  Qj=0 W  Qj_nominal_specify=off  Qj_nominal_value=1  Qj_nominal_unit=W  accumulatedSwitchingLosses_specify=off  accumulatedSwitchingLosses_priority=None  accumulatedSwitchingLosses=0 J
      settings: InternalSimscapePortConfiguration="{\"Bottom\":[],\"Left\":[{\"id\":\"G_elec\",\"label\":\"\",\"type\":\"foundation.electrical.electrical\"},{\"id\":\"H\",\"label\":\"\",\"type\":\"foundation.thermal.thermal\"}],\"Right\":[{\"id\":\"D\",\"label\":\"\",\"type\":\"foundation.electrical.electrical\"},{\"id\":\"S\",\"label\":\"\",\"type\":\"foundation.electrical.electrical\"}],\"Top\":[]}"
  G : PMIOPort  Side=Left
  thermal_port : PMIOPort  Port=2  Side=Left
  D : PMIOPort  Port=3  Side=Left
  S : PMIOPort  Port=4  Side=Right
  connections:
  G3R160MT17D/RConn1 -- Diode/RConn1 -- D/RConn1
  G3R160MT17D/RConn2 -- Diode/LConn1 -- S/RConn1
  G/RConn1 -- G3R160MT17D/LConn1
  G3R160MT17D/LConn2 -- thermal_port/RConn1

== system single_phase_multilevel/flying_capacitor_leg/switch_22/gate_driver ==
  cmd : Inport
  Controlled Voltage Source : fl_lib/Electrical/Electrical Sources/Controlled Voltage Source
  Diode1 : fl_lib/Electrical/Electrical Elements/Diode  Vf=0.6 V  Ron=0.3 Ohm  Goff=1e-8 1/Ohm  i_specify=off  i_priority=None  i=0 A  i_nominal_specify=off  i_nominal_value=1  i_nominal_unit=A  v_specify=off  v_priority=None  v=0 V  v_nominal_specify=off  v_nominal_value=1  v_nominal_unit=V
  Diode2 : fl_lib/Electrical/Electrical Elements/Diode  Vf=0.6 V  Ron=0.3 Ohm  Goff=1e-8 1/Ohm  i_specify=off  i_priority=None  i=0 A  i_nominal_specify=off  i_nominal_value=1  i_nominal_unit=A  v_specify=off  v_priority=None  v=0 V  v_nominal_specify=off  v_nominal_value=1  v_nominal_unit=V
  Resistor : fl_lib/Electrical/Electrical Elements/Resistor  R=Rg_on Ohm  i_specify=off  i_priority=None  i=0 A  i_nominal_specify=off  i_nominal_value=1  i_nominal_unit=A  v_specify=off  v_priority=None  v=0 V  v_nominal_specify=off  v_nominal_value=1  v_nominal_unit=V
  Resistor1 : fl_lib/Electrical/Electrical Elements/Resistor  R=Rg_off Ohm  i_specify=off  i_priority=None  i=0 A  i_nominal_specify=off  i_nominal_value=1  i_nominal_unit=A  v_specify=off  v_priority=None  v=0 V  v_nominal_specify=off  v_nominal_value=1  v_nominal_unit=V
  Simulink-PS Converter : nesl_utility/Simulink-PS Converter  PhysicalDomain=network_engine_domain  SubClassName=ps_input  LeftPortType=input  RightPortType=output  PseudoPeriodic=off  Frequencies=[]  NoiseDistribution=none  NoiseParameters=[]  Unit=V  AffineConversion=off  FilteringAndDerivatives=provide  SimscapeFilterOrder=1  InputFilterTimeConstant=0.001  UdotUserProvided=0
  gate : PMIOPort  Side=Right
  source : PMIOPort  Port=2  Side=Right
  wires:
  cmd/1 -> Simulink-PS Converter/1
  connections:
  Resistor/LConn1 -- Controlled Voltage Source/LConn1 -- Resistor1/LConn1
  Diode2/LConn1 -- Resistor/RConn1
  Controlled Voltage Source/RConn1 -- Simulink-PS Converter/RConn1
  Controlled Voltage Source/RConn2 -- source/RConn1
  Diode1/LConn1 -- gate/RConn1 -- Diode2/RConn1
  Diode1/RConn1 -- Resistor1/RConn1
